simulink model "FSM_Jacob"  (R2024b)
settings: Solver=FixedStepDiscrete  StartTime=0.0  StopTime=10.0  FixedStep=0.1  RelTol=1e-3  EnableMultiTasking=on
settings Model: Creator=jacob  LastModifiedBy=jacob
settings SolverCC: AlgebraicLoopSolver=TrustRegion  AutoInsertRateTranBlk=on
settings DataIOCC: LimitDataPoints=on
settings OptimizationCC: LifeSpan=inf
settings DebuggingCC: UnconnectedInputMsg=warning  UnconnectedOutputMsg=warning  UnconnectedLineMsg=warning  AllowSymbolicDim=off  SFUnexpectedBacktrackingDiag=warning  SFNoUnconditionalDefaultTransitionDiag=warning  SFExecutionAtInitializationDiag=none  ArithmeticOperatorsInVariantConditions=warning
settings ModelReferenceCC: EnableRefExpFcnMdlSchedulingChecks=on
settings SFSimCC: SimUseLocalCustomCode=off  CustomCodeUndefinedFunction=UseInterfaceOnly
settings RTWCC: RTWUseLocalCustomCode=off  GPUComputeCapability=3.5  DLArmComputeVersion=19.05
settings CodeAppCC: StateflowObjectComments=on
settings GRTTargetCC: TargetLangStandard=C89/C90 (ANSI)
settings ConfigComp: CovMetricSettings=dw  CovSaveCumulativeToWorkspaceVar=on  CovSaveSingleToWorkspaceVar=on  CovExternalEMLEnable=off

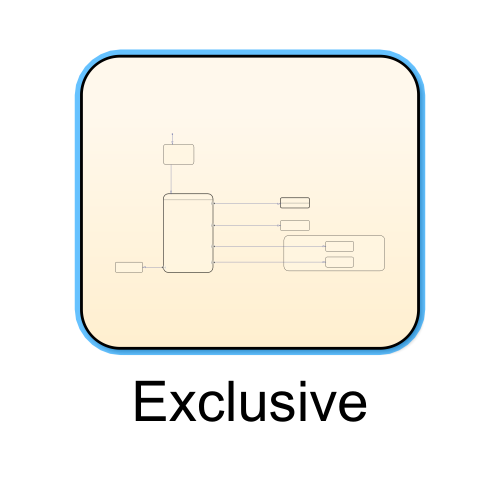
[thumbnail: Simulink's stored preview of the top-level diagram]
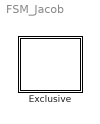
== system FSM_Jacob ==
  Exclusive : Stateflow chart  TreatAsAtomicUnit=on

== stateflow chart FSM_Jacob/Exclusive ==
  state Initialization
  state ObjectDetection
    state DetectObject
    state Rotate
    state IdentifyColor
    state EstimateObjLocation
    state NoObject
    state IdentifyGender
    state LocateCustomer
    DetectObject -> Rotate [order 1] : [class=='none']
    Rotate -> DetectObject
    (default) -> (junction 19)
    (junction 136) -> 135
    IdentifyColor -> IdentifyColor [order 1] : [color == 'red']
    (junction 19) -> DetectObject [order 1] : [obj]
    (junction 19) -> NoObject [order 2]
    DetectObject -> IdentifyColor [order 5] : [class=='traffic_light']
    IdentifyColor -> (junction 136) [order 2] : [color=='green']{goal='ingredients'}
    (junction 94) -> (junction 136)
    EstimateObjLocation -> (junction 94) [order 1] : [~inReach]
    DetectObject -> EstimateObjLocation [order 6] : [class=='bun']
    (junction 45) -> (junction 94)
    EstimateObjLocation -> 86 [order 2] : [inReach]
    DetectObject -> EstimateObjLocation [order 2] : [class=='patty']
    DetectObject -> IdentifyGender [order 4] : [class=='face']
    IdentifyGender -> (junction 69) : [genderIdentified]
    (junction 69) -> (junction 45) [order 1] : [image=='face']{goal='customer'}
    NoObject -> 120
    (junction 69) -> (junction 72) [order 2]
    (junction 74) -> (junction 45)
    LocateCustomer -> (junction 74) [order 1] : [~inReach]
    DetectObject -> 55 [order 3] : [class=='stop_sign']
    (junction 72) -> LocateCustomer : [image=='customer']
    LocateCustomer -> 116 [order 2] : [inReach]
    DetectObject -> 120 [order 7] : [timeout]
  state Navigation
    entry:
    goalReached=false;
    state PathPlanning
    state TrajectoryPlanning
    state TrajectoryExecution
    (default) -> PathPlanning
    TrajectoryExecution -> PathPlanning [order 1] : [~goalReached]
    PathPlanning -> TrajectoryPlanning
    TrajectoryPlanning -> TrajectoryExecution
    TrajectoryExecution -> 150 [order 2] : [goalReached]
  state TaskPlanning
  state Idle
  state ActuateGrasper
    state Pickup
    state Deposit
  state Error
  (default) -> Initialization
  Initialization -> ObjectDetection : {obj='traffic_light'}
  28 -> Navigation
  151 -> TaskPlanning
  56 -> Idle
  87 -> Pickup
  117 -> Deposit
  121 -> Error
